simulink model "model_19a"  (R2019a)
settings: Solver=ode4  StartTime=0.0  StopTime=tfinal  FixedStep=dt  RelTol=1e-3
values from neighbouring files (symbols this model uses):
  A_lateral = [YV , (W0+YP) , -U0+YR, g*cos(THETA0), 0, 0 ... (first row only)    [pre_simulink.m]
  A_longitudinal = [XU,XW,-W0,-g*cos(THETA0), 0, 0;         ZU/(1-ZWD),ZW/(1-ZWD),(ZQ+U0)/(1-ZWD),-g*sin(THETA0)/(1-ZWD), 0, 0;         MU+MWD*ZU/(1-ZWD),MW+MWD*ZW/(1-ZWD),MQ+MWD*(ZQ+U0)/(1-ZWD),-MWD*g*sin(THETA0)/(1-ZWD), 0, 0;         0,0,1,0, 0, 0 ... (first row only)    [pre_simulink.m]
  B_lateral = [YDA , YDR ... (first row only)    [pre_simulink.m]
  B_longitudinal = [XDE,XDTH ... (first row only)    [pre_simulink.m]
  C_lateral = eye(size(A_lateral))    [pre_simulink.m]
  C_longitudinal = eye(size(A_longitudinal))    [pre_simulink.m]
  Controls_Matrix = [0,    XDE,   XDTH,      0 ... (first row only)    [aircraft_data_reader.m]
  D_lateral = zeros(size(B_lateral))    [pre_simulink.m]
  D_longitudinal = zeros(size(B_longitudinal))    [pre_simulink.m]
  g = aircraft_data(52)    [aircraft_data_reader.m]
  Ixx = aircraft_data(53)    [aircraft_data_reader.m]
  Iyy = aircraft_data(54)    [aircraft_data_reader.m]
  Izz = aircraft_data(55)    [aircraft_data_reader.m]
  K_ElevFromPitch = tf(C1_ElevFromPitch).num{1}(1)    [pre_simulink.m]
  Kd_ElevFromPitch = tf(C2_ElevFromPitch).num{1}(1)    [pre_simulink.m]
  Ki_ElevFromPitch = tf(C1_ElevFromPitch).num{1}(2)    [pre_simulink.m]
  m = aircraft_data(51)    [aircraft_data_reader.m]
  mg0 = m*g * [ sin(s0(8)) ; -cos(s0(8))*sin(s0(7)) ; -cos(s0(8))*cos(s0(7)) ]    [aircraft_data_reader.m]
  P0 = s0(4)    [aircraft_data_reader.m]
  PHI0 = s0(7)    [aircraft_data_reader.m]
  PSI0 = s0(9)    [aircraft_data_reader.m]
  Q0 = s0(5)    [aircraft_data_reader.m]
  R0 = s0(6)    [aircraft_data_reader.m]
  States_Matrix = [XU,   0,   XW,    0,   0,   0,    0 ... (first row only)    [aircraft_data_reader.m]
  THETA0 = s0(8)    [aircraft_data_reader.m]
  Thrust0 = 0.5*rho*Vto^2*S*CD    [aircraft_data_reader.m]
  Thrustmax = 14800    [aircraft_data_reader.m]
  U0 = s0(1)    [aircraft_data_reader.m]
  V0 = s0(2)    [aircraft_data_reader.m]
  W0 = s0(3)    [aircraft_data_reader.m]
  X0 = 0    [aircraft_data_reader.m]
  Y0 = 0    [aircraft_data_reader.m]
  Z0 = -500    [aircraft_data_reader.m]
undefined symbols (not defined in the file or in its folder): A_lateral_1DOF, A_lateral_2DOF, A_lateral_3DOF_DR, A_lateral_3DOF_SP, A_longitudinal_lp, A_longitudinal_sp, alpha, B_lateral_1DOF, B_lateral_2DOF, B_lateral_3DOF_DR, B_lateral_3DOF_SP, B_longitudinal_lp, B_longitudinal_sp, beta, C_lateral_1DOF, C_lateral_2DOF, C_lateral_3DOF_DR, C_lateral_3DOF_SP, C_longitudinal_lp, C_longitudinal_sp, d_a, d_e, D_lateral_1DOF, D_lateral_2DOF, D_lateral_3DOF_DR, D_lateral_3DOF_SP, D_longitudinal_lp, D_longitudinal_sp, d_r, d_th, Earth, h_CMD, initial_states_bus, p, phi, phi_CMD, psi, psi_CMD, q, r, theta, theta_CMD, u_CMD, v, VT, w, wdot, WGS84, x, y, z
libraries: cstblocks x20, simulink_extras x12, SignalEditorBlockLib x6, dspsigops x3, shared6dof x1, aerolibasang x1, aerolibtransform2 x1, aerolibfltsims x1
settings Model: Creator=ahmed  LastModifiedBy=ahmed
settings DebuggingCC: SignalInfNanChecking=warning  CheckMatrixSingularityMsg=warning  SignalLabelMismatchMsg=warning  UnconnectedInputMsg=none  UnconnectedOutputMsg=none  UnconnectedLineMsg=none  StateNameClashWarn=warning
settings ModelReferenceCC: EnableRefExpFcnMdlSchedulingChecks=off
settings RTWCC: Description=Generic Real-Time Target

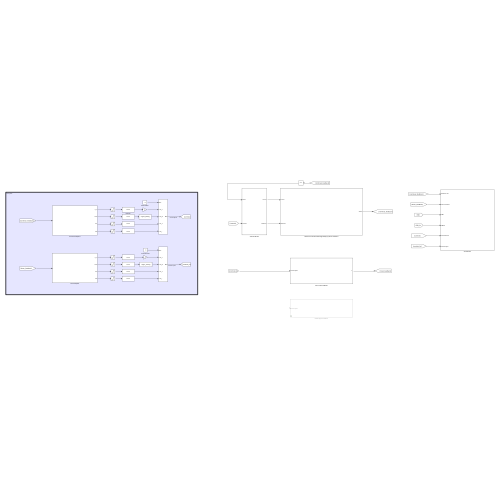
[thumbnail: Simulink's stored preview of the top-level diagram]
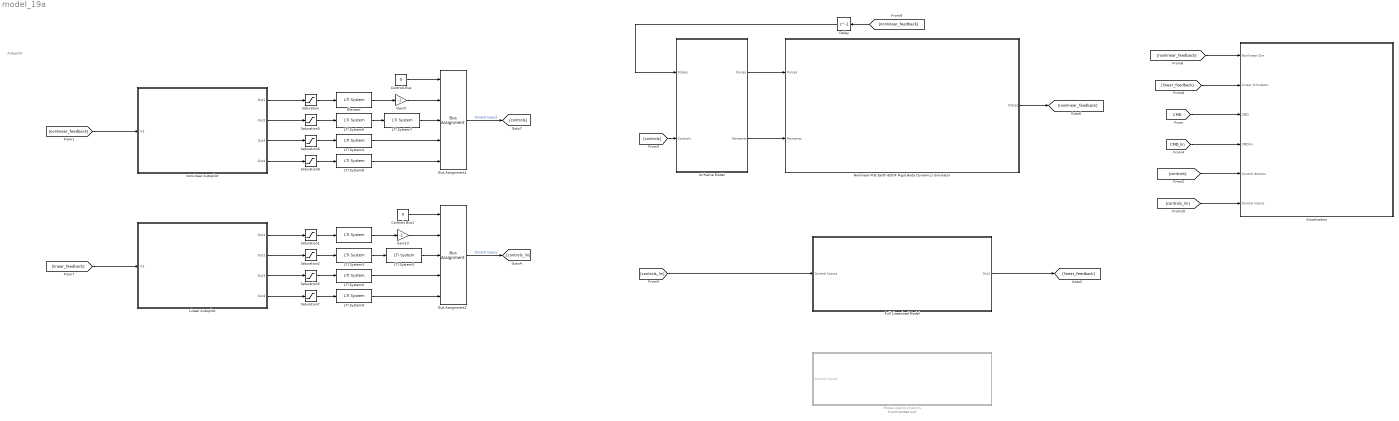
== system model_19a ==
  note: Autopilot
  " " : cstblocks/LTI System  sys=servo  IC=[]
  Airframe Model : Subsystem
  Bus Assignment1 : BusAssignment  AssignedSignals=d_e,d_th,d_a,d_r
  Bus Assignment2 : BusAssignment  AssignedSignals=d_e,d_th,d_a,d_r
  Controls Bus : Constant  Value=0  OutDataTypeStr=Bus: Controls_bus_T
  Controls Bus1 : Constant  Value=0  OutDataTypeStr=Bus: Lin_Controls_bus_T
  Delay : Delay  DelayLength=1  InitialCondition=initial_states_bus
  Elevator : cstblocks/LTI System  sys=servo  IC=[]
  Full Linearized Model : Subsystem
  Gain13 : Gain  Gain=-1
  Gain5 : Gain  Gain=-1
  LTI System{2..4,6,8..9} (6 alike) : cstblocks/LTI System  sys=servo  IC=[]
  LTI System5 : cstblocks/LTI System  sys=engine_timelag  IC=[]
  LTI System7 : cstblocks/LTI System  sys=engine_timelag  IC=[]
  Linear Autopilot : Subsystem
  Modes Approximations : Subsystem  Commented=on
  Nonlinear Flat Earth 6DOF Rigid Body Dynamics Simulator : Subsystem
  Saturation : Saturate  UpperLimit=30*pi/180  LowerLimit=-30*pi/180
  Saturation1 : Saturate  UpperLimit=30*pi/180  LowerLimit=-30*pi/180
  Saturation2 : Saturate  UpperLimit=Thrustmax - Thrust0  LowerLimit=3700 - Thrust0  LinearizeAsGain=off
  Saturation3 : Saturate  UpperLimit=Thrustmax - Thrust0  LowerLimit=3700 - Thrust0  LinearizeAsGain=off
  Saturation5 : Saturate  UpperLimit=50*pi/180  LowerLimit=-50*pi/180  LinearizeAsGain=off
  Saturation6 : Saturate  UpperLimit=50*pi/180  LowerLimit=-50*pi/180  LinearizeAsGain=off
  Saturation7 : Saturate  UpperLimit=15*pi/180  LowerLimit=-15*pi/180  LinearizeAsGain=off
  Saturation8 : Saturate  UpperLimit=15*pi/180  LowerLimit=-15*pi/180  LinearizeAsGain=off
  Visualization : Subsystem
  nonLinear Autopilot : Subsystem
  wires:
  Airframe Model/1(Forces) -> Nonlinear Flat Earth 6DOF Rigid Body Dynamics Simulator/1(Forces)
  Airframe Model/2(Moments) -> Nonlinear Flat Earth 6DOF Rigid Body Dynamics Simulator/2(Moments)
  Delay/1 -> Airframe Model/1(States)
  [CMD] -> Visualization/3(CMD)
  Bus Assignment1/1 -> [controls]  "Control Inputs"
  Controls Bus/1 -> Bus Assignment1/1
  Full Linearized Model/1(Out1) -> [linear_feedback]
  [linear_feedback] -> Visualization/2(Linear Simulator)
  Nonlinear Flat Earth 6DOF Rigid Body Dynamics Simulator/1(States) -> [nonlinear_feedback]
  [nonlinear_feedback] -> Visualization/1(Nonlinear Sim)
  [nonlinear_feedback] -> Delay/1
  LTI System6/1 -> LTI System7/1
  Saturation/1 -> Elevator/1
  LTI System7/1 -> Bus Assignment1/3
  Elevator/1 -> Gain5/1
  Saturation3/1 -> LTI System6/1
  Saturation6/1 -> LTI System4/1
  LTI System4/1 -> Bus Assignment1/4
  Saturation8/1 -> LTI System8/1
  LTI System8/1 -> Bus Assignment1/5
  [controls] -> Visualization/5(Control Actions)
  Gain5/1 -> Bus Assignment1/2
  [controls] -> Airframe Model/2(Controls)
  [controls_lin] -> Full Linearized Model/1(Control Inputs)
  LTI System5/1 -> Bus Assignment2/3
  LTI System9/1 -> Bus Assignment2/5
  LTI System3/1 -> LTI System5/1
  Gain13/1 -> Bus Assignment2/2
  LTI System2/1 -> Bus Assignment2/4
  " "/1 -> Gain13/1
  Saturation1/1 -> " "/1
  Saturation2/1 -> LTI System3/1
  Controls Bus1/1 -> Bus Assignment2/1
  Saturation5/1 -> LTI System2/1
  Bus Assignment2/1 -> [controls_lin]  "Control Inputs"
  Saturation7/1 -> LTI System9/1
  [linear_feedback] -> Linear Autopilot/1(In1)
  [nonlinear_feedback] -> nonLinear Autopilot/1(In1)
  [CMD_lin] -> Visualization/4(CMDlin)
  [controls_lin] -> Visualization/6(Control Inputs)
  Linear Autopilot/3(Out3) -> Saturation5/1
  Linear Autopilot/4(Out4) -> Saturation7/1
  nonLinear Autopilot/3(Out3) -> Saturation6/1
  nonLinear Autopilot/4(Out4) -> Saturation8/1
  nonLinear Autopilot/1(Out1) -> Saturation/1
  nonLinear Autopilot/2(Out2) -> Saturation3/1
  Linear Autopilot/1(Out1) -> Saturation1/1
  Linear Autopilot/2(Out2) -> Saturation2/1

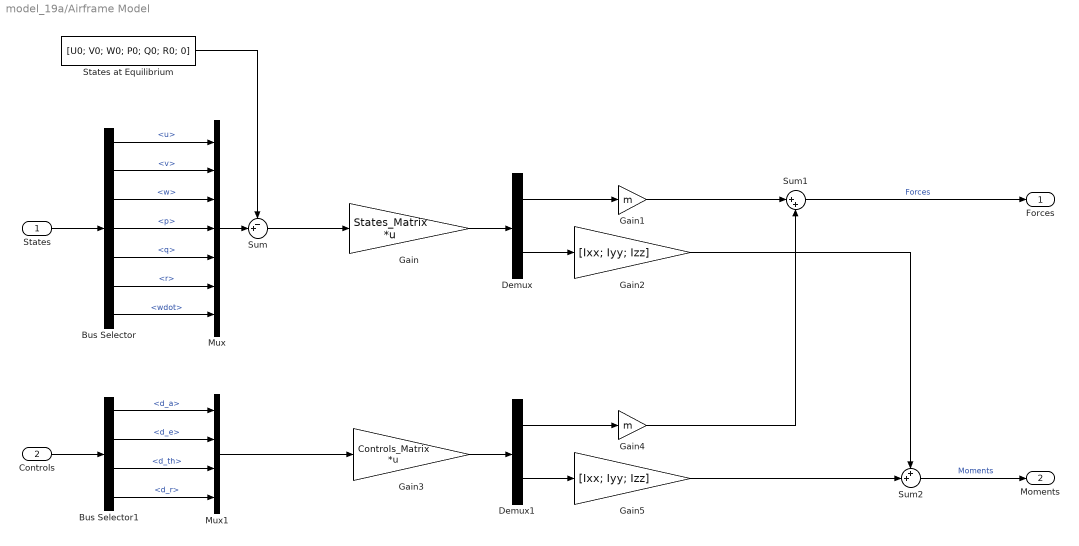
== system model_19a/Airframe Model ==
  States : Inport  OutDataTypeStr=Bus: States_bus_T
  Controls : Inport  Port=2  OutDataTypeStr=Bus: Controls_bus_T
  Bus Selector : BusSelector  OutputSignals=u,v,w,p,q,r,wdot
  Bus Selector1 : BusSelector  OutputSignals=d_a,d_e,d_th,d_r
  Demux : Demux  Outputs=2
  Demux1 : Demux  Outputs=2
  Gain : Gain  Gain=States_Matrix  Multiplication=Matrix(K*u)
  Gain1 : Gain  Gain=m
  Gain2 : Gain  Gain=[Ixx; Iyy; Izz]
  Gain3 : Gain  Gain=Controls_Matrix  Multiplication=Matrix(K*u)
  Gain4 : Gain  Gain=m
  Gain5 : Gain  Gain=[Ixx; Iyy; Izz]
  Mux : Mux  Inputs=7
  Mux1 : Mux
  States at Equilibrium : Constant  Value=[U0; V0; W0; P0; Q0; R0; 0]
  Sum : Sum  Inputs=-+|
  Sum1 : Sum  Inputs=|++
  Sum2 : Sum  Inputs=++|
  Forces : Outport
  Moments : Outport  Port=2
  wires:
  Sum1/1 -> Forces/1  "Forces"
  Sum2/1 -> Moments/1  "Moments"
  States/1 -> Bus Selector/1
  Bus Selector/2 -> Mux/2  "<v>"
  Bus Selector/1 -> Mux/1  "<u>"
  Bus Selector/3 -> Mux/3  "<w>"
  Bus Selector/4 -> Mux/4  "<p>"
  Bus Selector/5 -> Mux/5  "<q>"
  Bus Selector/6 -> Mux/6  "<r>"
  Bus Selector/7 -> Mux/7  "<wdot>"
  Mux/1 -> Sum/2
  States at Equilibrium/1 -> Sum/1
  Sum/1 -> Gain/1
  Gain/1 -> Demux/1
  Demux/1 -> Gain1/1
  Demux/2 -> Gain2/1
  Gain1/1 -> Sum1/1
  Gain2/1 -> Sum2/1
  Demux1/2 -> Gain5/1
  Gain3/1 -> Demux1/1
  Controls/1 -> Bus Selector1/1
  Bus Selector1/3 -> Mux1/3  "<d_th>"
  Bus Selector1/2 -> Mux1/2  "<d_e>"
  Bus Selector1/1 -> Mux1/1  "<d_a>"
  Bus Selector1/4 -> Mux1/4  "<d_r>"
  Mux1/1 -> Gain3/1
  Gain5/1 -> Sum2/2
  Demux1/1 -> Gain4/1
  Gain4/1 -> Sum1/2

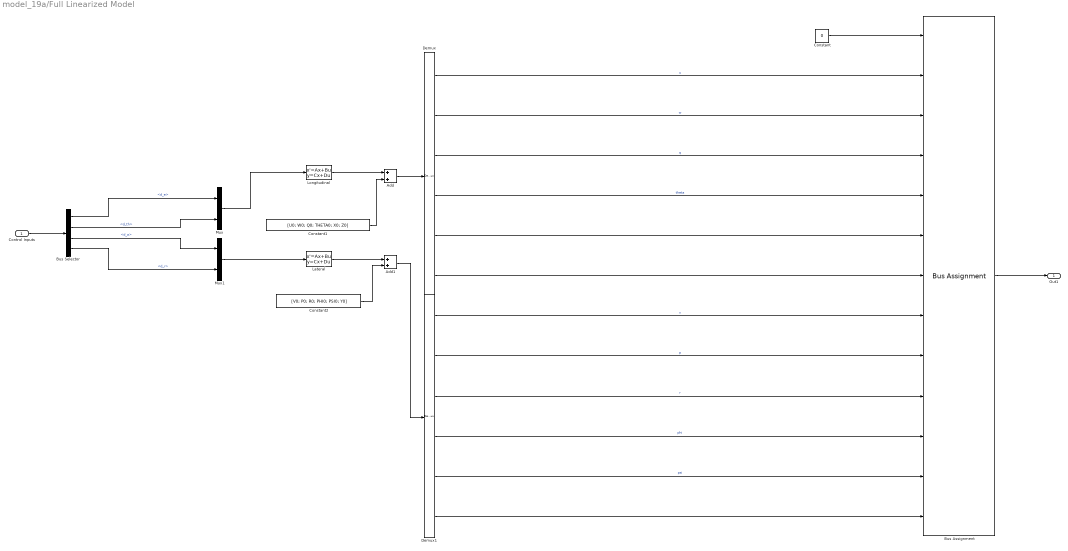
== system model_19a/Full Linearized Model ==
  Control Inputs : Inport
  Add : Sum
  Add1 : Sum
  Bus Assignment : BusAssignment  AssignedSignals=u,w,q,theta,x,z,v,p,r,phi,psi,y
  Bus Selector : BusSelector  OutputSignals=d_e,d_th,d_a,d_r
  Constant : Constant  Value=0  OutDataTypeStr=Bus: Lin_States_bus_T
  Constant1 : Constant  Value=[U0; W0; Q0; THETA0; X0; Z0]
  Constant2 : Constant  Value=[V0; P0; R0; PHI0; PSI0; Y0]
  Demux : Demux  Outputs=6
  Demux1 : Demux  Outputs=6
  Lateral : StateSpace  A=A_lateral  B=B_lateral  C=C_lateral  D=D_lateral  InitialCondition=0
  Longitudinal : StateSpace  A=A_longitudinal  B=B_longitudinal  C=C_longitudinal  D=D_longitudinal  InitialCondition=0
  Mux : Mux  Inputs=2
  Mux1 : Mux  Inputs=2
  Out1 : Outport
  wires:
  Bus Selector/4 -> Mux1/2  "<d_r>"
  Bus Selector/1 -> Mux/1  "<d_e>"
  Bus Selector/2 -> Mux/2  "<d_th>"
  Mux/1 -> Longitudinal/1
  Bus Selector/3 -> Mux1/1  "<d_a>"
  Longitudinal/1 -> Add/1
  Control Inputs/1 -> Bus Selector/1
  Demux1/2 -> Bus Assignment/9  "p"
  Demux1/1 -> Bus Assignment/8  "v"
  Demux/4 -> Bus Assignment/5  "theta"
  Demux/2 -> Bus Assignment/3  "w"
  Demux/3 -> Bus Assignment/4  "q"
  Demux1/3 -> Bus Assignment/10  "r"
  Demux/1 -> Bus Assignment/2  "u"
  Demux1/4 -> Bus Assignment/11  "phi"
  Bus Assignment/1 -> Out1/1
  Mux1/1 -> Lateral/1
  Constant/1 -> Bus Assignment/1
  Demux1/5 -> Bus Assignment/12  "psi"
  Add/1 -> Demux/1
  Constant1/1 -> Add/2
  Constant2/1 -> Add1/2
  Lateral/1 -> Add1/1
  Add1/1 -> Demux1/1
  Demux/5 -> Bus Assignment/6
  Demux/6 -> Bus Assignment/7
  Demux1/6 -> Bus Assignment/13

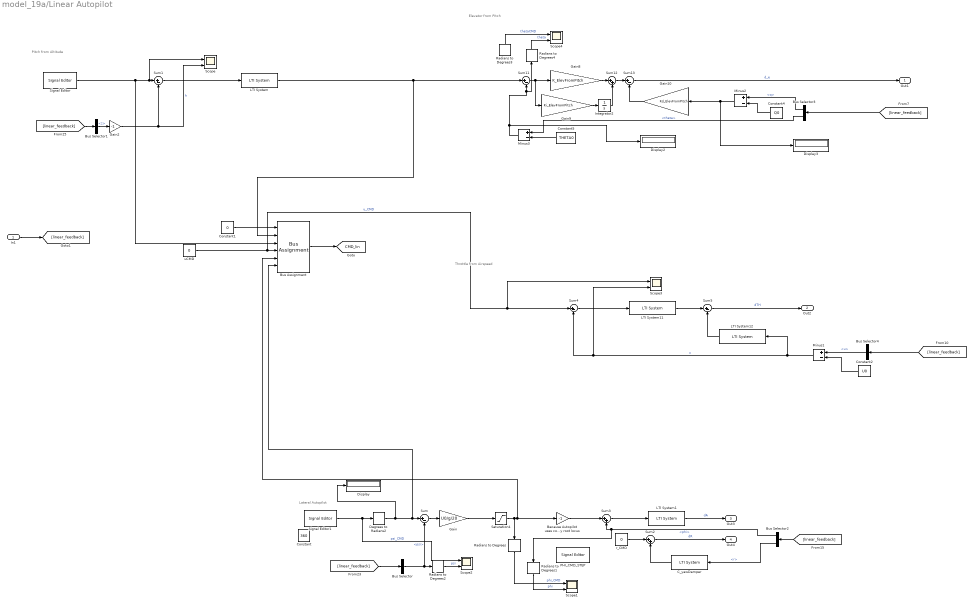
== system model_19a/Linear Autopilot ==
  note: Pitch from Altitude
  note: Elevator from Pitch
  note: Throttle from Airspeed
  note: Lateral Autopilot
  In1 : Inport
  Because Autopilot uses complemetary root locus : Gain  Gain=-1
  Bus Assignment : BusAssignment  AssignedSignals=theta_CMD,h_CMD,u_CMD,phi_CMD,psi_CMD
  Bus Selector : BusSelector  OutputSignals=psi
  Bus Selector1 : BusSelector  OutputSignals=z
  Bus Selector2 : BusSelector  OutputSignals=phi,r
  Bus Selector3 : BusSelector  OutputSignals=q,theta
  Bus Selector4 : BusSelector  OutputSignals=u
  C_yawDamper : cstblocks/LTI System  sys=C_yawDamper  IC=[]
  Constant : Constant  Value=360
  Constant1 : Constant  Value=0  OutDataTypeStr=Bus: CMDlin_States_bus_T
  Constant2 : Constant  Value=U0
  Constant4 : Constant  Value=Q0
  Constant5 : Constant  Value=THETA0
  Degrees to Radians2 : simulink_extras/Transformations/Degrees to Radians
  Display : Display
  Display2 : Display
  Display3 : Display
  Gain : Gain  Gain=U0/g/20
  Gain10 : Gain  Gain=Kd_ElevFromPitch
  Gain2 : Gain  Gain=-1
  Gain8 : Gain  Gain=K_ElevFromPitch
  Gain9 : Gain  Gain=Ki_ElevFromPitch
  Integrator2 : Integrator
  LTI System : cstblocks/LTI System  sys=C1_PitchFromAltitude  IC=[]
  LTI System1 : cstblocks/LTI System  sys=C1_AileronFromRoll  IC=[]
  LTI System11 : cstblocks/LTI System  sys=C1_ThrottleFromAirspeed  IC=[]
  LTI System12 : cstblocks/LTI System  sys=C2_ThrottleFromAirspeed  IC=[]
  Minus1 : Sum  Inputs=+-
  Minus2 : Sum  Inputs=+-
  Minus3 : Sum  Inputs=+-
  PHI_CMD_STEP : SignalEditorBlockLib/Signal Editor  FileName=some_signal.mat  ActiveScenario=Scenario  ActiveSignal=Signal 1  IsBus=off  OutputBusObjectStr=Bus: BusObject  SampleTime=0  Interpolate=off  ZeroCross=off  OutputAfterFinalValue=Setting to zero  Unit=inherit  PreserveSignalName=on
  Radians to Degrees{,1..4} (5 alike) : simulink_extras/Transformations/Radians to Degrees
  Saturation4 : Saturate  UpperLimit=35*pi/180  LowerLimit=-35*pi/180
  Scope{,1..4} (5 alike) : Scope  NumInputPorts=2
  Signal Editor : SignalEditorBlockLib/Signal Editor  FileName=hCMD.mat  ActiveScenario=Mission  ActiveSignal=h_CMD  IsBus=off  OutputBusObjectStr=Bus: BusObject  SampleTime=0  Interpolate=off  ZeroCross=off  OutputAfterFinalValue=Setting to zero  Unit=inherit  PreserveSignalName=on
  Signal Editor1 : SignalEditorBlockLib/Signal Editor  FileName=psiCMD.mat  ActiveScenario=Mission  ActiveSignal=psi_CMD  IsBus=off  OutputBusObjectStr=Bus: BusObject  SampleTime=0  Interpolate=off  ZeroCross=off  OutputAfterFinalValue=Setting to zero  Unit=inherit  PreserveSignalName=on
  Sum{,1,4..5,11,13} (6 alike) : Sum  Inputs=|+-
  Sum12 : Sum  Inputs=|++
  Sum2 : Sum  Inputs=|++
  Sum3 : Sum  Inputs=|++
  r_CMD : Constant  Value=0
  uCMD : Constant  Value=0
  Out1 : Outport
  Out2 : Outport  Port=2
  Out3 : Outport  Port=3
  Out4 : Outport  Port=4
  tag scope: CMD_lin=global
  wires:
  Bus Selector3/2 -> Minus3/1  "<theta>"
  Gain10/1 -> Sum13/2
  Bus Assignment/1 -> [CMD_lin]
  Gain8/1 -> Sum12/1
  Because Autopilot uses complemetary root locus/1 -> Sum3/1
  Radians to Degrees2/1 -> Scope2/2  "psi"
  Sum12/1 -> Sum13/1
  C_yawDamper/1 -> Sum2/2
  Constant5/1 -> Minus3/2
  Minus1/1 -> LTI System12/1, Scope3/2, Sum4/2  "u"
  Minus2/1 -> Display3/1, Gain10/1
  Bus Selector2/2 -> C_yawDamper/1  "<r>"
  Sum2/1 -> Out4/1  "dR"
  Sum5/1 -> Out2/1  "dTH"
  Radians to Degrees3/1 -> Scope4/1  "thetaCMD"
  Degrees to Radians2/1 -> Display/1, Bus Assignment/6, Sum/1
  Signal Editor1/1 -> Scope2/1, Degrees to Radians2/1  "psi_CMD"
  [linear_feedback] -> Bus Selector1/1
  Bus Selector1/1 -> Gain2/1  "<z>"
  Gain9/1 -> Integrator2/1
  Bus Selector3/1 -> Minus2/1  "<q>"
  [linear_feedback] -> Bus Selector3/1
  LTI System12/1 -> Sum5/2
  Bus Selector4/1 -> Minus1/1  "<u>"
  Sum/1 -> Gain/1
  Constant4/1 -> Minus2/2
  LTI System11/1 -> Sum5/1
  Radians to Degrees4/1 -> Scope4/2  "theta"
  Saturation4/1 -> Because Autopilot uses complemetary root locus/1, Bus Assignment/5, Radians to Degrees/1
  Sum1/1 -> LTI System/1
  Signal Editor/1 -> Bus Assignment/3, Scope/1, Sum1/1
  Sum3/1 -> LTI System1/1
  Sum13/1 -> Out1/1  "d_e"
  Constant2/1 -> Minus1/2
  Minus3/1 -> Display2/1, Radians to Degrees4/1, Sum11/2
  [linear_feedback] -> Bus Selector2/1
  Constant1/1 -> Bus Assignment/1
  LTI System1/1 -> Out3/1  "dA"
  Bus Selector2/1 -> Radians to Degrees1/1, Sum3/2  "<phi>"
  Integrator2/1 -> Sum12/2
  Gain2/1 -> Sum1/2, Scope/2  "h"
  Gain/1 -> Saturation4/1
  Sum11/1 -> Gain9/1, Gain8/1
  Radians to Degrees1/1 -> Scope1/2  "phi"
  [linear_feedback] -> Bus Selector/1
  r_CMD/1 -> Sum2/1
  Sum4/1 -> LTI System11/1
  [linear_feedback] -> Bus Selector4/1
  uCMD/1 -> Sum4/1, Scope3/1, Bus Assignment/4  "u_CMD"
  Bus Selector/1 -> Radians to Degrees2/1, Sum/2  "<psi>"
  Radians to Degrees/1 -> Scope1/1  "phi_CMD"
  In1/1 -> [linear_feedback]
  LTI System/1 -> Sum11/1, Bus Assignment/2

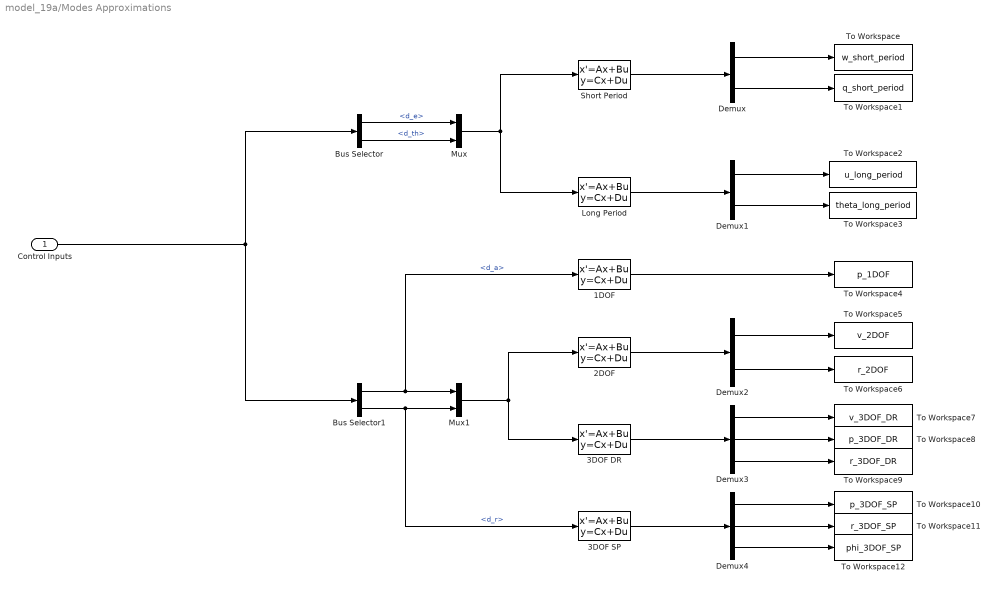
== system model_19a/Modes Approximations ==
  Control Inputs : Inport
  1DOF : StateSpace  A=A_lateral_1DOF  B=B_lateral_1DOF  C=C_lateral_1DOF  D=D_lateral_1DOF  InitialCondition=0
  2DOF : StateSpace  A=A_lateral_2DOF  B=B_lateral_2DOF  C=C_lateral_2DOF  D=D_lateral_2DOF  InitialCondition=0
  3DOF DR : StateSpace  A=A_lateral_3DOF_DR  B=B_lateral_3DOF_DR  C=C_lateral_3DOF_DR  D=D_lateral_3DOF_DR  InitialCondition=0
  3DOF SP : StateSpace  A=A_lateral_3DOF_SP  B=B_lateral_3DOF_SP  C=C_lateral_3DOF_SP  D=D_lateral_3DOF_SP  InitialCondition=0
  Bus Selector : BusSelector  OutputSignals=d_e,d_th
  Bus Selector1 : BusSelector  OutputSignals=d_a,d_r
  Demux : Demux  Outputs=2
  Demux1 : Demux  Outputs=2
  Demux2 : Demux  Outputs=2
  Demux3 : Demux  Outputs=3
  Demux4 : Demux  Outputs=3
  Long Period : StateSpace  A=A_longitudinal_lp  B=B_longitudinal_lp  C=C_longitudinal_lp  D=D_longitudinal_lp  InitialCondition=0
  Mux : Mux  Inputs=2
  Mux1 : Mux  Inputs=2
  Short Period : StateSpace  A=A_longitudinal_sp  B=B_longitudinal_sp  C=C_longitudinal_sp  D=D_longitudinal_sp  InitialCondition=0
  To Workspace : ToWorkspace  VariableName=w_short_period  SaveFormat=Timeseries  SampleTime=-1
  To Workspace1 : ToWorkspace  VariableName=q_short_period  SaveFormat=Timeseries  SampleTime=-1
  To Workspace10 : ToWorkspace  VariableName=p_3DOF_SP  SaveFormat=Timeseries  SampleTime=-1
  To Workspace11 : ToWorkspace  VariableName=r_3DOF_SP  SaveFormat=Timeseries  SampleTime=-1
  To Workspace12 : ToWorkspace  VariableName=phi_3DOF_SP  SaveFormat=Timeseries  SampleTime=-1
  To Workspace2 : ToWorkspace  VariableName=u_long_period  SaveFormat=Timeseries  SampleTime=-1
  To Workspace3 : ToWorkspace  VariableName=theta_long_period  SaveFormat=Timeseries  SampleTime=-1
  To Workspace4 : ToWorkspace  VariableName=p_1DOF  SaveFormat=Timeseries  SampleTime=-1
  To Workspace5 : ToWorkspace  VariableName=v_2DOF  SaveFormat=Timeseries  SampleTime=-1
  To Workspace6 : ToWorkspace  VariableName=r_2DOF  SaveFormat=Timeseries  SampleTime=-1
  To Workspace7 : ToWorkspace  VariableName=v_3DOF_DR  SaveFormat=Timeseries  SampleTime=-1
  To Workspace8 : ToWorkspace  VariableName=p_3DOF_DR  SaveFormat=Timeseries  SampleTime=-1
  To Workspace9 : ToWorkspace  VariableName=r_3DOF_DR  SaveFormat=Timeseries  SampleTime=-1
  wires:
  Demux4/2 -> To Workspace11/1
  Bus Selector1/1 -> 1DOF/1, Mux1/1  "<d_a>"
  Demux1/1 -> To Workspace2/1
  Demux3/2 -> To Workspace8/1
  Demux3/3 -> To Workspace9/1
  Demux2/1 -> To Workspace5/1
  Demux2/2 -> To Workspace6/1
  3DOF SP/1 -> Demux4/1
  Mux1/1 -> 3DOF DR/1, 2DOF/1
  Short Period/1 -> Demux/1
  Demux3/1 -> To Workspace7/1
  Demux4/1 -> To Workspace10/1
  Demux1/2 -> To Workspace3/1
  Control Inputs/1 -> Bus Selector/1, Bus Selector1/1
  Long Period/1 -> Demux1/1
  Demux4/3 -> To Workspace12/1
  1DOF/1 -> To Workspace4/1
  Bus Selector1/2 -> 3DOF SP/1, Mux1/2  "<d_r>"
  3DOF DR/1 -> Demux3/1
  Demux/1 -> To Workspace/1
  2DOF/1 -> Demux2/1
  Bus Selector/2 -> Mux/2  "<d_th>"
  Mux/1 -> Long Period/1, Short Period/1
  Demux/2 -> To Workspace1/1
  Bus Selector/1 -> Mux/1  "<d_e>"

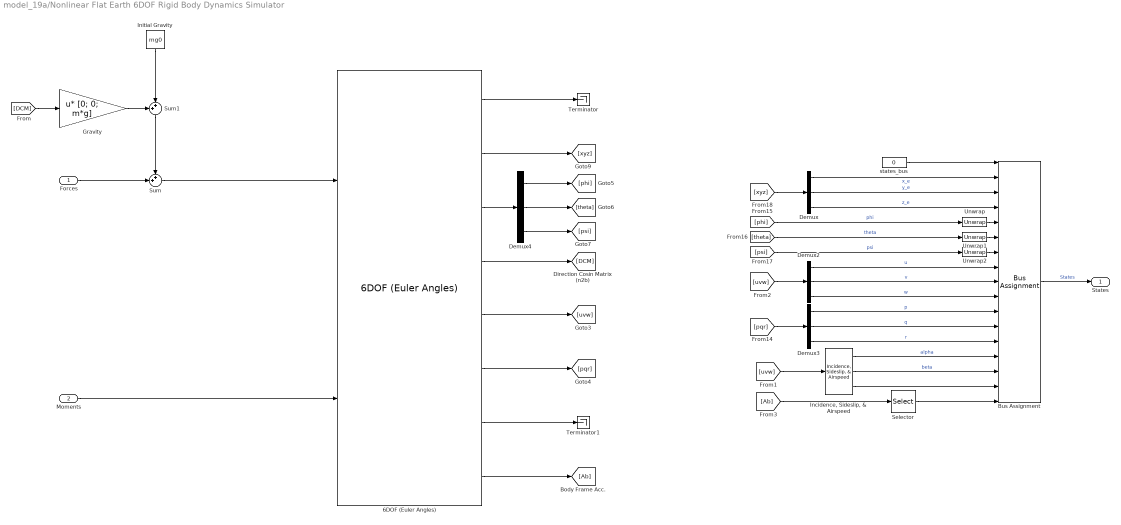
== system model_19a/Nonlinear Flat Earth 6DOF Rigid Body Dynamics Simulator ==
  Forces : Inport
  Moments : Inport  Port=2
  6DOF (Euler Angles) : shared6dof/6DOF (Euler Angles)  units=English (Velocity in ft/s)  mtype=Fixed  rep=Euler Angles  xme_0=[X0, Y0, Z0]  Vm_0=[U0, V0, W0]  eul_0=[PHI0, THETA0, PSI0]  pm_0=[P0, Q0, R0]  mass_0=m  mass_e=0.5  mass_f=2.0  inertia=I  inertia_e=eye(3)  inertia_f=2*eye(3)  k_quat=1.0  vre_flag=on  abi_flag=off  aMode=0  xme_statename=''  Vm_statename=''  eul_statename=''  quat_statename=''  pm_statename=''  mass_statename=''
  Bus Assignment : BusAssignment  AssignedSignals=x,y,z,phi,theta,psi,u,v,w,p,q,r,alpha,beta,VT,wdot
  Demux{,2..4} (4 alike) : Demux  Outputs=3
  Gravity : Gain  Gain=[0; 0; m*g]  Multiplication=Matrix(u*K)
  "Incidence, Sideslip, & Airspeed" : aerolibasang/Incidence, Sideslip, & Airspeed
  Initial Gravity : Constant  Value=mg0
  Selector : Selector  InputPortWidth=3  IndexOptions=Index vector (dialog)  Indices=3  OutputSizes=1
  Sum : Sum  Inputs=++|
  Sum1 : Sum  Inputs=++|
  Terminator : Terminator
  Terminator1 : Terminator
  Unwrap : dspsigops/Unwrap  tol=pi  running=off
  Unwrap1 : dspsigops/Unwrap  tol=pi  running=off
  Unwrap2 : dspsigops/Unwrap  tol=pi  running=off
  states_bus : Constant  Value=0  OutDataTypeStr=Bus: States_bus_T  SampleTime=-1
  States : Outport  OutDataTypeStr=Bus: States_bus_T
  wires:
  Bus Assignment/1 -> States/1  "States"
  [theta] -> Unwrap1/1  "theta"
  Demux3/2 -> Bus Assignment/12  "q"
  states_bus/1 -> Bus Assignment/1
  Forces/1 -> Sum/2
  [pqr] -> Demux3/1
  Demux2/2 -> Bus Assignment/9  "v"
  [psi] -> Unwrap2/1  "psi"
  Demux3/3 -> Bus Assignment/13  "r"
  Demux2/1 -> Bus Assignment/8  "u"
  Demux2/3 -> Bus Assignment/10  "w"
  [xyz] -> Demux/1
  Demux/3 -> Bus Assignment/4  "z_e"
  [phi] -> Unwrap/1  "phi"
  Demux/2 -> Bus Assignment/3  "y_e"
  Demux/1 -> Bus Assignment/2  "x_e"
  Demux3/1 -> Bus Assignment/11  "p"
  Unwrap/1 -> Bus Assignment/5
  Unwrap1/1 -> Bus Assignment/6
  Unwrap2/1 -> Bus Assignment/7
  [DCM] -> Gravity/1
  Gravity/1 -> Sum1/1
  Initial Gravity/1 -> Sum1/2
  Sum1/1 -> Sum/1
  [uvw] -> "Incidence, Sideslip, & Airspeed"/1
  "Incidence, Sideslip, & Airspeed"/3 -> Bus Assignment/16
  "Incidence, Sideslip, & Airspeed"/2 -> Bus Assignment/15  "beta"
  "Incidence, Sideslip, & Airspeed"/1 -> Bus Assignment/14  "alpha"
  [uvw] -> Demux2/1
  [Ab] -> Selector/1
  Selector/1 -> Bus Assignment/17
  Sum/1 -> 6DOF (Euler Angles)/1
  Demux4/1 -> [phi]
  6DOF (Euler Angles)/3 -> Demux4/1
  Demux4/2 -> [theta]
  Demux4/3 -> [psi]
  6DOF (Euler Angles)/8 -> [Ab]
  6DOF (Euler Angles)/5 -> [uvw]
  6DOF (Euler Angles)/4 -> [DCM]
  Moments/1 -> 6DOF (Euler Angles)/2
  6DOF (Euler Angles)/6 -> [pqr]
  6DOF (Euler Angles)/2 -> [xyz]
  6DOF (Euler Angles)/1 -> Terminator/1
  6DOF (Euler Angles)/7 -> Terminator1/1

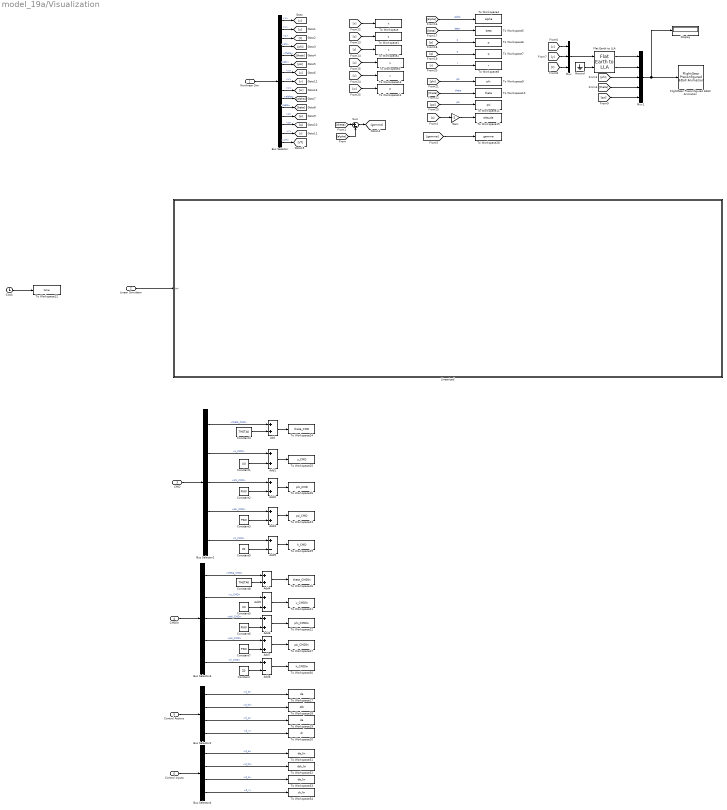
== system model_19a/Visualization ==
  Nonlinear Sim : Inport
  Linear Simulator : Inport  Port=2
  CMD : Inport  Port=3
  CMDlin : Inport  Port=4
  Control Actions : Inport  Port=5
  Control Inputs : Inport  Port=6
  Add{,1..7} (8 alike) : Sum
  Add8 : Sum  Inputs=+-
  Add9 : Sum  Inputs=+-
  Bus Selector : BusSelector  OutputSignals=x,y,z,phi,theta,psi,u,v,w,alpha,beta,p,q,r,VT
  Bus Selector1 : BusSelector  OutputSignals=theta_CMD,u_CMD,phi_CMD,psi_CMD,h_CMD
  Bus Selector2 : BusSelector  OutputSignals=d_e,d_th,d_a,d_r
  Bus Selector3 : BusSelector  OutputSignals=theta_CMD,u_CMD,phi_CMD,psi_CMD,h_CMD
  Bus Selector4 : BusSelector  OutputSignals=d_e,d_th,d_a,d_r
  Clock : Clock
  Constant : Constant  Value=Z0
  Constant1 : Constant  Value=U0
  Constant2 : Constant  Value=PHI0
  Constant3 : Constant  Value=PSI0
  Constant4 : Constant  Value=THETA0
  Constant5 : Constant  Value=U0
  Constant6 : Constant  Value=PHI0
  Constant7 : Constant  Value=PSI0
  Constant8 : Constant  Value=THETA0
  Constant9 : Constant  Value=Z0
  Display : Display
  Flat Earth to LLA : aerolibtransform2/Flat Earth to LLA  units=English  ptype=Earth (WGS84)  F=1/298.257223563  R=20925646.3255  LL0=[19.718, -155.054]  psi=90
  FlightGear Preconfigured 6DoF Animation : aerolibfltsims/FlightGear Preconfigured 6DoF Animation  xFlightGearVersion=v2019.1  DestinationIpAddress=127.0.0.1  DestinationPort=5501  SampleTime=0.02  packetVersion=24
  Gain : Gain  Gain=-1
  Ground : Ground
  Linearized : Subsystem
  Mux : Mux  Inputs=3
  Mux1 : Mux  Inputs=5
  Sum : Sum  Inputs=|+-
  To Workspace : ToWorkspace  VariableName=x  SaveFormat=Timeseries  SampleTime=-1
  To Workspace1 : ToWorkspace  VariableName=y  SaveFormat=Timeseries  SampleTime=-1
  To Workspace10 : ToWorkspace  VariableName=theta  SaveFormat=Timeseries  SampleTime=-1
  To Workspace11 : ToWorkspace  VariableName=psi  SaveFormat=Timeseries  SampleTime=-1
  To Workspace12 : ToWorkspace  VariableName=time  SaveFormat=Timeseries  SampleTime=-1
  To Workspace13 : ToWorkspace  VariableName=v  SaveFormat=Timeseries  SampleTime=-1
  To Workspace14 : ToWorkspace  VariableName=w  SaveFormat=Timeseries  SampleTime=-1
  To Workspace15 : ToWorkspace  VariableName=altitude  SaveFormat=Timeseries  SampleTime=-1
  To Workspace16 : ToWorkspace  VariableName=theta_CMDlin  SaveFormat=Timeseries  SampleTime=-1
  To Workspace17 : ToWorkspace  VariableName=de  SaveFormat=Timeseries  SampleTime=-1
  To Workspace18 : ToWorkspace  VariableName=dth  SaveFormat=Timeseries  SampleTime=-1
  To Workspace19 : ToWorkspace  VariableName=da  SaveFormat=Timeseries  SampleTime=-1
  To Workspace2 : ToWorkspace  VariableName=z  SaveFormat=Timeseries  SampleTime=-1
  To Workspace20 : ToWorkspace  VariableName=dr  SaveFormat=Timeseries  SampleTime=-1
  To Workspace21 : ToWorkspace  VariableName=u_CMDlin  SaveFormat=Timeseries  SampleTime=-1
  To Workspace22 : ToWorkspace  VariableName=phi_CMDlin  SaveFormat=Timeseries  SampleTime=-1
  To Workspace23 : ToWorkspace  VariableName=psi_CMD  SaveFormat=Timeseries  SampleTime=-1
  To Workspace24 : ToWorkspace  VariableName=theta_CMD  SaveFormat=Timeseries  SampleTime=-1
  To Workspace25 : ToWorkspace  VariableName=u_CMD  SaveFormat=Timeseries  SampleTime=-1
  To Workspace26 : ToWorkspace  VariableName=phi_CMD  SaveFormat=Timeseries  SampleTime=-1
  To Workspace27 : ToWorkspace  VariableName=psi_CMDlin  SaveFormat=Timeseries  SampleTime=-1
  To Workspace28 : ToWorkspace  VariableName=gamma  SaveFormat=Timeseries  SampleTime=-1
  To Workspace29 : ToWorkspace  VariableName=h_CMD  SaveFormat=Timeseries  SampleTime=-1
  To Workspace3 : ToWorkspace  VariableName=u  SaveFormat=Timeseries  SampleTime=-1
  To Workspace30 : ToWorkspace  VariableName=h_CMDlin  SaveFormat=Timeseries  SampleTime=-1
  To Workspace31 : ToWorkspace  VariableName=de_lin  SaveFormat=Timeseries  SampleTime=-1
  To Workspace32 : ToWorkspace  VariableName=dth_lin  SaveFormat=Timeseries  SampleTime=-1
  To Workspace33 : ToWorkspace  VariableName=da_lin  SaveFormat=Timeseries  SampleTime=-1
  To Workspace34 : ToWorkspace  VariableName=dr_lin  SaveFormat=Timeseries  SampleTime=-1
  To Workspace4 : ToWorkspace  VariableName=alpha  SaveFormat=Timeseries  SampleTime=-1
  To Workspace5 : ToWorkspace  VariableName=beta  SaveFormat=Timeseries  SampleTime=-1
  To Workspace6 : ToWorkspace  VariableName=p  SaveFormat=Timeseries  SampleTime=-1
  To Workspace7 : ToWorkspace  VariableName=q  SaveFormat=Timeseries  SampleTime=-1
  To Workspace8 : ToWorkspace  VariableName=r  SaveFormat=Timeseries  SampleTime=-1
  To Workspace9 : ToWorkspace  VariableName=phi  SaveFormat=Timeseries  SampleTime=-1
  wires:
  Bus Selector/6 -> [psi]  "<psi>"
  Bus Selector/1 -> [x]  "<x>"
  Bus Selector/7 -> [u]  "<u>"
  Bus Selector/4 -> [phi]  "<phi>"
  Bus Selector/10 -> [alpha]  "<alpha>"
  Bus Selector/14 -> [r]  "<r>"
  Bus Selector/11 -> [beta]  "<beta>"
  Bus Selector/5 -> [theta]  "<theta>"
  Bus Selector/13 -> [q]  "<q>"
  Bus Selector/12 -> [p]  "<p>"
  Bus Selector/2 -> [y]  "<y>"
  Bus Selector/3 -> [z]  "<z>"
  Nonlinear Sim/1 -> Bus Selector/1
  [x] -> To Workspace/1
  [y] -> To Workspace1/1
  [z] -> To Workspace2/1
  [u] -> To Workspace3/1
  Clock/1 -> To Workspace12/1
  [phi] -> To Workspace9/1  "phi"
  [theta] -> To Workspace10/1  "theta"
  [psi] -> To Workspace11/1  "psi"
  [alpha] -> To Workspace4/1  "alpha"
  [beta] -> To Workspace5/1  "beta"
  [p] -> To Workspace6/1  "p"
  [q] -> To Workspace7/1  "q"
  [r] -> To Workspace8/1  "r"
  [v] -> To Workspace13/1
  Bus Selector/8 -> [v]  "<v>"
  Bus Selector/9 -> [w]  "<w>"
  [w] -> To Workspace14/1
  [theta] -> Sum/1
  [alpha] -> Sum/2
  Sum/1 -> [gamma]
  Bus Selector/15 -> [VT]  "<VT>"
  Gain/1 -> To Workspace15/1
  Linear Simulator/1 -> Linearized/1(In4)
  CMD/1 -> Bus Selector1/1
  Bus Selector1/1 -> Add/1  "<theta_CMD>"
  Control Actions/1 -> Bus Selector2/1
  Bus Selector1/2 -> Add1/1  "<u_CMD>"
  Add/1 -> To Workspace24/1
  Constant4/1 -> Add/2
  Constant1/1 -> Add1/2
  Add1/1 -> To Workspace25/1
  Constant2/1 -> Add2/2
  Bus Selector1/3 -> Add2/1  "<phi_CMD>"
  Add2/1 -> To Workspace26/1
  Add3/1 -> To Workspace23/1
  Constant3/1 -> Add3/2
  Bus Selector1/4 -> Add3/1  "<psi_CMD>"
  Bus Selector2/1 -> To Workspace17/1  "<d_e>"
  Bus Selector2/2 -> To Workspace18/1  "<d_th>"
  Bus Selector2/3 -> To Workspace19/1  "<d_a>"
  Bus Selector2/4 -> To Workspace20/1  "<d_r>"
  Constant7/1 -> Add7/2
  Bus Selector3/1 -> Add4/1  "<theta_CMD>"
  Bus Selector3/4 -> Add7/1  "<psi_CMD>"
  Constant8/1 -> Add4/2
  Add7/1 -> To Workspace27/1
  CMDlin/1 -> Bus Selector3/1
  Add6/1 -> To Workspace22/1
  Bus Selector3/3 -> Add6/1  "<phi_CMD>"
  Bus Selector3/2 -> Add5/1  "<u_CMD>"
  Constant6/1 -> Add6/2
  Add5/1 -> To Workspace21/1
  Constant5/1 -> Add5/2
  Add4/1 -> To Workspace16/1
  [gamma] -> To Workspace28/1
  [z] -> Gain/1
  Constant/1 -> Add8/2
  Add8/1 -> To Workspace30/1
  Bus Selector3/5 -> Add8/1  "<h_CMD>"
  Constant9/1 -> Add9/2
  Add9/1 -> To Workspace29/1
  Bus Selector1/5 -> Add9/1  "<h_CMD>"
  Ground/1 -> Flat Earth to LLA/2
  [x] -> Mux/1
  [y] -> Mux/2
  [z] -> Mux/3
  Mux/1 -> Flat Earth to LLA/1
  Flat Earth to LLA/1 -> Mux1/1
  Flat Earth to LLA/2 -> Mux1/2
  Bus Selector4/4 -> To Workspace34/1  "<d_r>"
  Bus Selector4/2 -> To Workspace32/1  "<d_th>"
  Bus Selector4/1 -> To Workspace31/1  "<d_e>"
  Bus Selector4/3 -> To Workspace33/1  "<d_a>"
  Control Inputs/1 -> Bus Selector4/1
  [phi] -> Mux1/3
  [theta] -> Mux1/4
  [psi] -> Mux1/5
  Mux1/1 -> Display/1, FlightGear Preconfigured 6DoF Animation/1

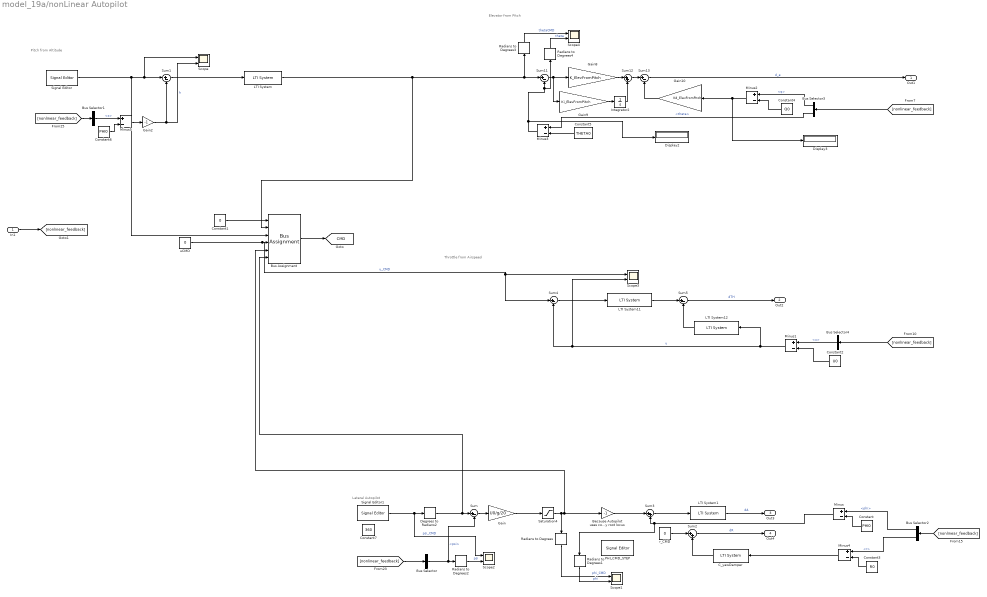
== system model_19a/nonLinear Autopilot ==
  note: Pitch from Altitude
  note: Elevator from Pitch
  note: Throttle from Airspeed
  note: Lateral Autopilot
  In1 : Inport
  Because Autopilot uses complemetary root locus : Gain  Gain=-1
  Bus Assignment : BusAssignment  AssignedSignals=theta_CMD,h_CMD,u_CMD,phi_CMD,psi_CMD
  Bus Selector : BusSelector  OutputSignals=psi
  Bus Selector1 : BusSelector  OutputSignals=z
  Bus Selector2 : BusSelector  OutputSignals=phi,r
  Bus Selector3 : BusSelector  OutputSignals=q,theta
  Bus Selector4 : BusSelector  OutputSignals=u
  C_yawDamper : cstblocks/LTI System  sys=C_yawDamper  IC=[]
  Constant : Constant  Value=PHI0
  Constant1 : Constant  Value=0  OutDataTypeStr=Bus: CMD_States_bus_T
  Constant2 : Constant  Value=U0
  Constant3 : Constant  Value=R0
  Constant4 : Constant  Value=Q0
  Constant5 : Constant  Value=THETA0
  Constant6 : Constant  Value=PHI0
  Constant7 : Constant  Value=360
  Degrees to Radians2 : simulink_extras/Transformations/Degrees to Radians
  Display2 : Display
  Display3 : Display
  Gain : Gain  Gain=U0/g/20
  Gain10 : Gain  Gain=Kd_ElevFromPitch
  Gain2 : Gain  Gain=-1
  Gain8 : Gain  Gain=K_ElevFromPitch
  Gain9 : Gain  Gain=Ki_ElevFromPitch
  Integrator2 : Integrator
  LTI System : cstblocks/LTI System  sys=C1_PitchFromAltitude  IC=[]
  LTI System1 : cstblocks/LTI System  sys=C1_AileronFromRoll  IC=[]
  LTI System11 : cstblocks/LTI System  sys=C1_ThrottleFromAirspeed  IC=[]
  LTI System12 : cstblocks/LTI System  sys=C2_ThrottleFromAirspeed  IC=[]
  Minus{,1..5} (6 alike) : Sum  Inputs=+-
  PHI_CMD_STEP : SignalEditorBlockLib/Signal Editor  FileName=some_signal.mat  ActiveScenario=Scenario  ActiveSignal=Signal 1  IsBus=off  OutputBusObjectStr=Bus: BusObject  SampleTime=0  Interpolate=off  ZeroCross=off  OutputAfterFinalValue=Setting to zero  Unit=inherit  PreserveSignalName=on
  Radians to Degrees{,1..4} (5 alike) : simulink_extras/Transformations/Radians to Degrees
  Saturation4 : Saturate  UpperLimit=35*pi/180  LowerLimit=-35*pi/180
  Scope{,1..4} (5 alike) : Scope  NumInputPorts=2
  Signal Editor : SignalEditorBlockLib/Signal Editor  FileName=hCMD.mat  ActiveScenario=Mission  ActiveSignal=h_CMD  IsBus=off  OutputBusObjectStr=Bus: BusObject  SampleTime=0  Interpolate=off  ZeroCross=off  OutputAfterFinalValue=Setting to zero  Unit=inherit  PreserveSignalName=on
  Signal Editor1 : SignalEditorBlockLib/Signal Editor  FileName=psiCMD.mat  ActiveScenario=Mission  ActiveSignal=psi_CMD  IsBus=off  OutputBusObjectStr=Bus: BusObject  SampleTime=0  Interpolate=off  ZeroCross=off  OutputAfterFinalValue=Setting to zero  Unit=inherit  PreserveSignalName=on
  Sum{,1,4..5,11,13} (6 alike) : Sum  Inputs=|+-
  Sum12 : Sum  Inputs=|++
  Sum2 : Sum  Inputs=|++
  Sum3 : Sum  Inputs=|++
  r_CMD : Constant  Value=0
  uCMD : Constant  Value=0
  Out1 : Outport
  Out2 : Outport  Port=2
  Out3 : Outport  Port=3
  Out4 : Outport  Port=4
  tag scope: CMD=global
  wires:
  Bus Selector3/2 -> Minus3/1  "<theta>"
  Gain10/1 -> Sum13/2
  Bus Assignment/1 -> [CMD]
  Gain8/1 -> Sum12/1
  Because Autopilot uses complemetary root locus/1 -> Sum3/1
  Radians to Degrees2/1 -> Scope2/2  "psi"
  Sum12/1 -> Sum13/1
  C_yawDamper/1 -> Sum2/2
  Constant5/1 -> Minus3/2
  Minus1/1 -> LTI System12/1, Scope3/2, Sum4/2  "u"
  Minus2/1 -> Display3/1, Gain10/1
  Minus4/1 -> C_yawDamper/1
  Sum2/1 -> Out4/1  "dR"
  Sum5/1 -> Out2/1  "dTH"
  Radians to Degrees3/1 -> Scope4/1  "thetaCMD"
  Degrees to Radians2/1 -> Bus Assignment/6, Sum/1
  Signal Editor1/1 -> Scope2/1, Degrees to Radians2/1  "psi_CMD"
  [nonlinear_feedback] -> Bus Selector1/1
  Bus Selector1/1 -> Minus5/1  "<z>"
  Gain9/1 -> Integrator2/1
  Bus Selector3/1 -> Minus2/1  "<q>"
  [nonlinear_feedback] -> Bus Selector3/1
  LTI System12/1 -> Sum5/2
  Bus Selector4/1 -> Minus1/1  "<u>"
  Sum/1 -> Gain/1
  Constant4/1 -> Minus2/2
  LTI System11/1 -> Sum5/1
  Radians to Degrees4/1 -> Scope4/2  "theta"
  Saturation4/1 -> Because Autopilot uses complemetary root locus/1, Bus Assignment/5, Radians to Degrees/1
  Sum1/1 -> LTI System/1
  Signal Editor/1 -> Bus Assignment/3, Scope/1, Sum1/1
  Sum3/1 -> LTI System1/1
  Sum13/1 -> Out1/1  "d_e"
  Constant2/1 -> Minus1/2
  Minus3/1 -> Display2/1, Radians to Degrees4/1, Sum11/2
  [nonlinear_feedback] -> Bus Selector2/1
  Constant1/1 -> Bus Assignment/1
  LTI System1/1 -> Out3/1  "dA"
  Minus/1 -> Radians to Degrees1/1, Sum3/2
  Integrator2/1 -> Sum12/2
  Gain2/1 -> Sum1/2, Scope/2  "h"
  Gain/1 -> Saturation4/1
  Sum11/1 -> Gain9/1, Gain8/1
  Radians to Degrees1/1 -> Scope1/2  "phi"
  [nonlinear_feedback] -> Bus Selector/1
  r_CMD/1 -> Sum2/1
  Sum4/1 -> LTI System11/1
  [nonlinear_feedback] -> Bus Selector4/1
  uCMD/1 -> Sum4/1, Scope3/1, Bus Assignment/4  "u_CMD"
  Bus Selector/1 -> Radians to Degrees2/1, Sum/2  "<psi>"
  Radians to Degrees/1 -> Scope1/1  "phi_CMD"
  In1/1 -> [nonlinear_feedback]
  Bus Selector2/1 -> Minus/1  "<phi>"
  Constant/1 -> Minus/2
  Constant3/1 -> Minus4/2
  Bus Selector2/2 -> Minus4/1  "<r>"
  Constant6/1 -> Minus5/2
  Minus5/1 -> Gain2/1
  LTI System/1 -> Bus Assignment/2, Sum11/1, Radians to Degrees3/1

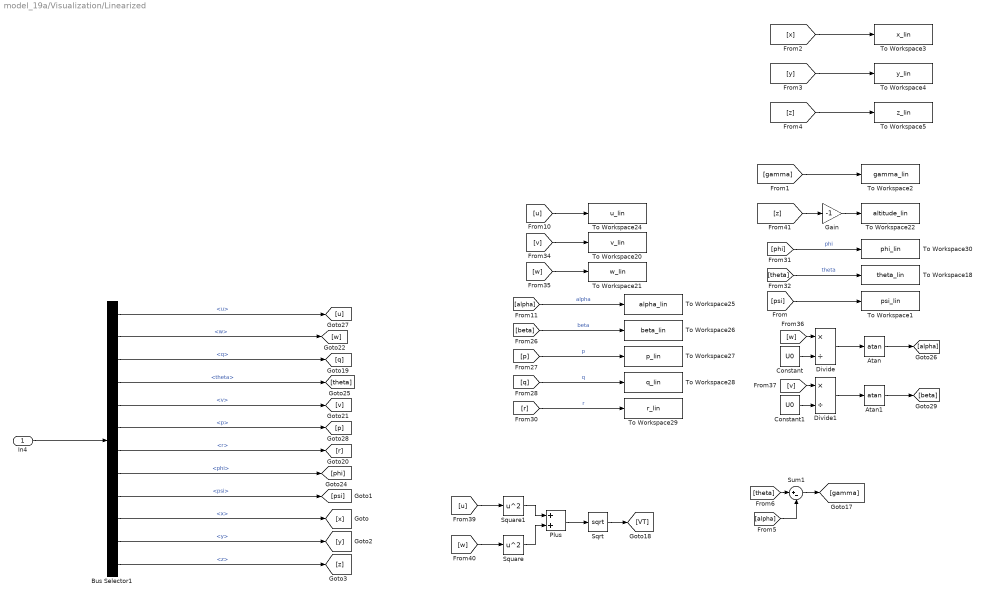
== system model_19a/Visualization/Linearized ==
  In4 : Inport
  Atan : Trigonometry  Operator=atan
  Atan1 : Trigonometry  Operator=atan
  Bus Selector1 : BusSelector  OutputSignals=u,w,q,theta,v,p,r,phi,psi,x,y,z
  Constant : Constant  Value=U0
  Constant1 : Constant  Value=U0
  Divide : Product  Inputs=*/
  Divide1 : Product  Inputs=*/
  Gain : Gain  Gain=-1
  Plus : Sum
  Sqrt : Sqrt  SaturateOnIntegerOverflow=on
  Square : Math  Operator=square  SaturateOnIntegerOverflow=on
  Square1 : Math  Operator=square  SaturateOnIntegerOverflow=on
  Sum1 : Sum  Inputs=|+-
  To Workspace1 : ToWorkspace  VariableName=psi_lin  SaveFormat=Timeseries  SampleTime=-1
  To Workspace18 : ToWorkspace  VariableName=theta_lin  SaveFormat=Timeseries  SampleTime=-1
  To Workspace2 : ToWorkspace  VariableName=gamma_lin  SaveFormat=Timeseries  SampleTime=-1
  To Workspace20 : ToWorkspace  VariableName=v_lin  SaveFormat=Timeseries  SampleTime=-1
  To Workspace21 : ToWorkspace  VariableName=w_lin  SaveFormat=Timeseries  SampleTime=-1
  To Workspace22 : ToWorkspace  VariableName=altitude_lin  SaveFormat=Timeseries  SampleTime=-1
  To Workspace24 : ToWorkspace  VariableName=u_lin  SaveFormat=Timeseries  SampleTime=-1
  To Workspace25 : ToWorkspace  VariableName=alpha_lin  SaveFormat=Timeseries  SampleTime=-1
  To Workspace26 : ToWorkspace  VariableName=beta_lin  SaveFormat=Timeseries  SampleTime=-1
  To Workspace27 : ToWorkspace  VariableName=p_lin  SaveFormat=Timeseries  SampleTime=-1
  To Workspace28 : ToWorkspace  VariableName=q_lin  SaveFormat=Timeseries  SampleTime=-1
  To Workspace29 : ToWorkspace  VariableName=r_lin  SaveFormat=Timeseries  SampleTime=-1
  To Workspace3 : ToWorkspace  VariableName=x_lin  SaveFormat=Timeseries  SampleTime=-1
  To Workspace30 : ToWorkspace  VariableName=phi_lin  SaveFormat=Timeseries  SampleTime=-1
  To Workspace4 : ToWorkspace  VariableName=y_lin  SaveFormat=Timeseries  SampleTime=-1
  To Workspace5 : ToWorkspace  VariableName=z_lin  SaveFormat=Timeseries  SampleTime=-1
  wires:
  [u] -> Square1/1
  [alpha] -> To Workspace25/1  "alpha"
  [r] -> To Workspace29/1  "r"
  [alpha] -> Sum1/2
  Sqrt/1 -> [VT]
  Constant/1 -> Divide/2
  [w] -> Divide/1
  Atan/1 -> [alpha]
  [p] -> To Workspace27/1  "p"
  [w] -> To Workspace21/1
  [beta] -> To Workspace26/1  "beta"
  Atan1/1 -> [beta]
  [v] -> Divide1/1
  [q] -> To Workspace28/1  "q"
  Plus/1 -> Sqrt/1
  [theta] -> To Workspace18/1  "theta"
  [z] -> Gain/1
  Divide/1 -> Atan/1
  In4/1 -> Bus Selector1/1
  Square/1 -> Plus/2
  Constant1/1 -> Divide1/2
  Square1/1 -> Plus/1
  [v] -> To Workspace20/1
  Divide1/1 -> Atan1/1
  [w] -> Square/1
  [phi] -> To Workspace30/1  "phi"
  [u] -> To Workspace24/1
  Sum1/1 -> [gamma]
  [theta] -> Sum1/1
  Bus Selector1/8 -> [phi]  "<phi>"
  Bus Selector1/4 -> [theta]  "<theta>"
  Bus Selector1/7 -> [r]  "<r>"
  Bus Selector1/3 -> [q]  "<q>"
  Bus Selector1/6 -> [p]  "<p>"
  Bus Selector1/2 -> [w]  "<w>"
  Bus Selector1/5 -> [v]  "<v>"
  Bus Selector1/1 -> [u]  "<u>"
  Bus Selector1/9 -> [psi]  "<psi>"
  [psi] -> To Workspace1/1
  [gamma] -> To Workspace2/1
  Bus Selector1/10 -> [x]  "<x>"
  Bus Selector1/11 -> [y]  "<y>"
  Bus Selector1/12 -> [z]  "<z>"
  Gain/1 -> To Workspace22/1
  [x] -> To Workspace3/1
  [y] -> To Workspace4/1
  [z] -> To Workspace5/1
